simulink model "OrbitFollowing"  (R2015b)
settings: Solver=VariableStepAuto  StartTime=0.0  StopTime=1000  FixedStep=0.01  RelTol=1e-4
values from neighbouring files (symbols this model uses):
  alpha = 1.65    [BeardMethod.m]    (also in OrbitCenter.m = abs((ang1-ang2)/2); RevisedMethod.m)
  course_int = course_int+2*pi    (= 6.28318530718)    [BeardMethod.m]    (also in RevisedMethod.m = -0.785398163397)
  cx = C(1)    [BeardMethod.m]    (also in RevisedMethod.m = 50)
  cy = C(2)    [BeardMethod.m]    (also in RevisedMethod.m = 50)
  d_int = norm([x.data(end),y.data(end)]-[cx,cy])    [BeardMethod.m]    (also in RevisedMethod.m = 15)
  epsi = 0.1    [BeardMethod.m]    (also in RevisedMethod.m = 0.5)
  gamma_end = (pi+(pi/2-2*alpha))    [OrbitCenter.m]    (also in RevisedMethod.m = 47.1238898038)
  gamma_int = atan2((y.data(end)-cy),(x.data(end)-cx))    [BeardMethod.m]    (also in RevisedMethod.m = 0.785398163397)
  j = Rotation(i)    [BeardMethod.m]    (also in RevisedMethod.m = -1)
  k = 0.02    [BeardMethod.m]    (also in RevisedMethod.m = 0.1)
  kk = pi/2    (= 1.57079632679)    [BeardMethod.m]    (also in RevisedMethod.m)
  phiw = 230/180*pi    (= 4.01425727959)    [BeardMethod.m]    (also in RevisedMethod.m)
  R = 10    [BeardMethod.m]    (also in RevisedMethod.m)
  Va = 13    [BeardMethod.m]    (also in RevisedMethod.m)
  w = 0.9    [BeardMethod.m]
libraries: simulink x1
settings Model: Creator=Bingyu Zhou  LastModifiedBy=Bingyu Zhou

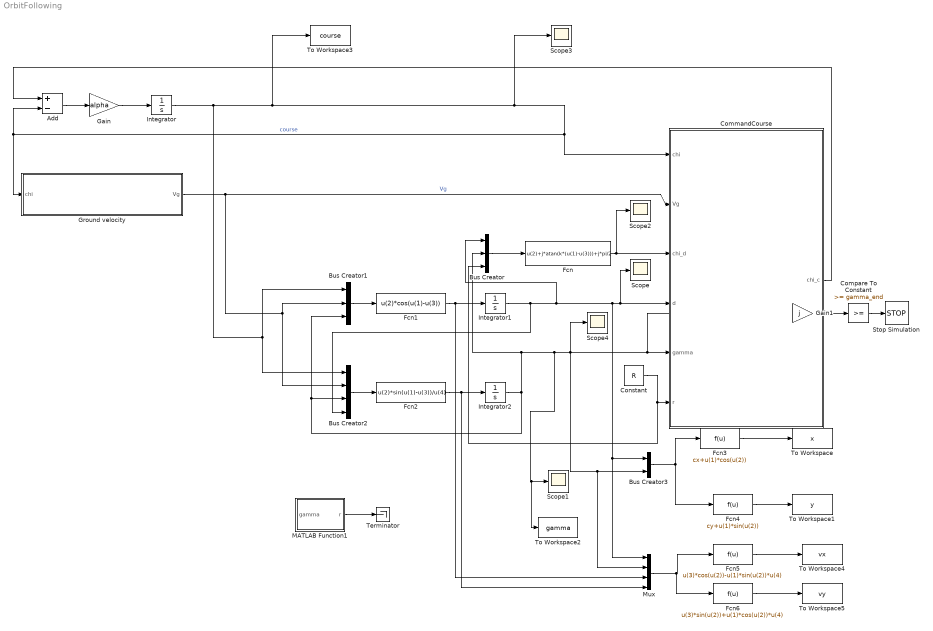
== system OrbitFollowing ==
  Add : Sum  Inputs=+-
  Bus Creator : BusCreator  Inputs=3
  Bus Creator1 : BusCreator  Inputs=3
  Bus Creator2 : BusCreator  Inputs=4
  Bus Creator3 : BusCreator  Inputs=2
  CommandCourse : Subsystem
  Compare To Constant : simulink/Logic and Bit Operations/Compare To Constant  relop=>=  const=gamma_end  OutDataTypeStr=boolean
  Constant : Constant  Value=R
  Fcn : Fcn  Expr=u(2)+j*atan(k*(u(1)-u(3)))+j*pi/2
  Fcn1 : Fcn  Expr=u(2)*cos(u(1)-u(3))
  Fcn2 : Fcn  Expr=u(2)*sin(u(1)-u(3))/u(4)
  Fcn3 : Fcn  Expr=cx+u(1)*cos(u(2))
  Fcn4 : Fcn  Expr=cy+u(1)*sin(u(2))
  Fcn5 : Fcn  Expr=u(3)*cos(u(2))-u(1)*sin(u(2))*u(4)
  Fcn6 : Fcn  Expr=u(3)*sin(u(2))+u(1)*cos(u(2))*u(4)
  Gain : Gain  Gain=alpha
  Gain1 : Gain  Gain=j
  Ground velocity : Subsystem
  Integrator : Integrator  InitialCondition=course_int
  Integrator1 : Integrator  InitialCondition=d_int
  Integrator2 : Integrator  InitialCondition=gamma_int
  MATLAB Function1 : MATLAB Function  TreatAsAtomicUnit=on
  Mux : Mux
  Scope{,1..4} (5 alike) : Scope
  Stop Simulation : Stop
  Terminator : Terminator
  To Workspace : ToWorkspace  VariableName=x  SaveFormat=Timeseries  SampleTime=-1
  To Workspace1 : ToWorkspace  VariableName=y  SaveFormat=Timeseries  SampleTime=-1
  To Workspace2 : ToWorkspace  VariableName=gamma  SaveFormat=Timeseries  SampleTime=-1
  To Workspace3 : ToWorkspace  VariableName=course  SaveFormat=Timeseries  SampleTime=-1
  To Workspace4 : ToWorkspace  VariableName=vx  SaveFormat=Timeseries  SampleTime=-1
  To Workspace5 : ToWorkspace  VariableName=vy  SaveFormat=Timeseries  SampleTime=-1
  wires:
  Add/1 -> Gain/1
  Gain/1 -> Integrator/1
  Integrator/1 -> To Workspace3/1, Scope3/1, CommandCourse/1(chi), Ground velocity/1(chi), Add/2, Bus Creator2/1, Bus Creator1/1  "course"
  Ground velocity/1(Vg) -> Bus Creator1/2, Bus Creator2/2, CommandCourse/2(Vg)  "Vg"
  Bus Creator/1 -> Fcn/1
  Bus Creator1/1 -> Fcn1/1
  Fcn1/1 -> Mux/3, Integrator1/1
  Integrator2/1 -> Bus Creator2/3, Bus Creator1/3, To Workspace2/1, Scope1/1, Scope4/1, Mux/2, Bus Creator3/2, Gain1/1, CommandCourse/5(gamma), Bus Creator/2
  Bus Creator2/1 -> Fcn2/1
  Integrator1/1 -> Bus Creator2/4, Bus Creator/1, Mux/1, Bus Creator3/1, Scope/1, CommandCourse/4(d)
  Fcn/1 -> Scope2/1, CommandCourse/3(chi_d)
  Bus Creator3/1 -> Fcn4/1, Fcn3/1
  Fcn3/1 -> To Workspace/1
  Fcn4/1 -> To Workspace1/1
  CommandCourse/1(chi_c) -> Add/1
  Constant/1 -> Bus Creator/3, CommandCourse/6("r ")
  MATLAB Function1/1(r) -> Terminator/1
  Compare To Constant/1 -> Stop Simulation/1
  Gain1/1 -> Compare To Constant/1
  Mux/1 -> Fcn6/1, Fcn5/1
  Fcn5/1 -> To Workspace4/1
  Fcn6/1 -> To Workspace5/1
  Fcn2/1 -> Mux/4, Integrator2/1

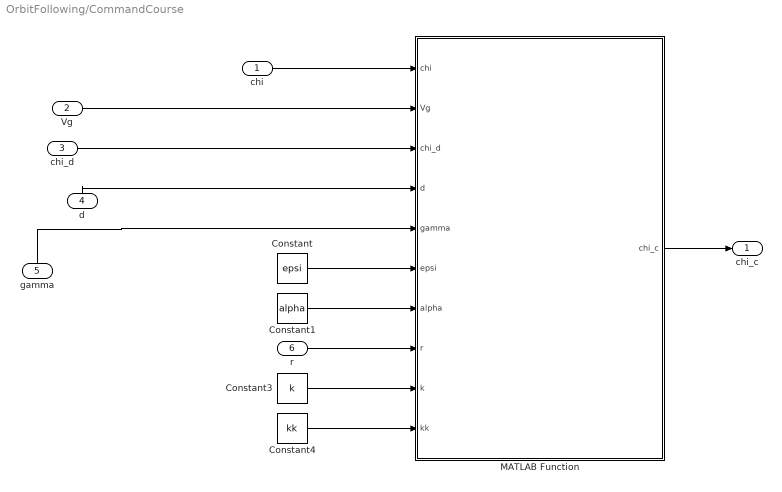
== system OrbitFollowing/CommandCourse ==
  chi : Inport
  Vg : Inport  Port=2
  chi_d : Inport  Port=3
  d : Inport  Port=4
  gamma : Inport  Port=5
  "r " : Inport  Port=6
  Constant : Constant  Value=epsi
  Constant1 : Constant  Value=alpha
  Constant3 : Constant  Value=k
  Constant4 : Constant  Value=kk
  MATLAB Function : MATLAB Function  TreatAsAtomicUnit=on
  chi_c : Outport
  wires:
  Constant/1 -> MATLAB Function/6(epsi)
  Constant1/1 -> MATLAB Function/7(alpha)
  Constant3/1 -> MATLAB Function/9(k)
  Constant4/1 -> MATLAB Function/10(kk)
  chi_d/1 -> MATLAB Function/3(chi_d)
  gamma/1 -> MATLAB Function/5(gamma)
  Vg/1 -> MATLAB Function/2(Vg)
  chi/1 -> MATLAB Function/1(chi)
  d/1 -> MATLAB Function/4(d)
  MATLAB Function/1(chi_c) -> chi_c/1
  "r "/1 -> MATLAB Function/8(r)

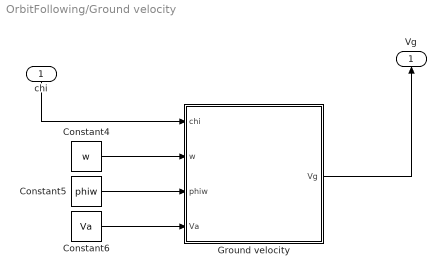
== system OrbitFollowing/Ground velocity ==
  chi : Inport
  Constant4 : Constant  Value=w
  Constant5 : Constant  Value=phiw
  Constant6 : Constant  Value=Va
  Ground velocity : MATLAB Function  TreatAsAtomicUnit=on
  Vg : Outport
  wires:
  Ground velocity/1(Vg) -> Vg/1
  chi/1 -> Ground velocity/1(chi)
  Constant6/1 -> Ground velocity/4(Va)
  Constant5/1 -> Ground velocity/3(phiw)
  Constant4/1 -> Ground velocity/2(w)

== matlab function OrbitFollowing/Ground velocity/Ground velocity ==
  data: chi input; Vg output; w input; phiw input; Va input
function Vg = GroundVelocity(chi,w,phiw,Va)
%generate the ground velocity based on course angle
Vg=w*cos(chi-phiw)+sqrt(Va^2-w^2*(sin(chi-phiw))^2);
end

== matlab function OrbitFollowing/CommandCourse/MATLAB Function ==
  data: chi input; chi_c output; Vg input; chi_d input; d input; gamma input; epsi input; alpha input; r input; k input; kk input
function chi_c = CommandCourse(chi,Vg,chi_d,d,gamma,epsi,alpha,r,k,kk)
%generate course angle for orbit following
sat=(chi-chi_d)/epsi;
if abs(sat)<=1
    rho=sat;
else
    rho=sign(sat);
end
beta=k/(1+(k*(d-r))^2);
chi_c=chi+Vg/alpha/d*sin(chi-gamma)-beta/alpha*Vg*cos(chi-gamma)-kk/alpha*rho;
end

== matlab function OrbitFollowing/MATLAB Function1 ==
  data: gamma input; r output
function r = radius(gamma)
%#codegen
if abs(gamma)<=4*pi
    r=70;
else
    r=50;
end
end
